simulink library "sim_model_lib"  (R2016b)
settings: Solver=ode45  StartTime=0.0  StopTime=10.0  RelTol=1e-3  EnableMultiTasking=on
libraries: env_environment_model_lib x1, mlp_mid_level_processor_lib x1, veh_vehicle_model_lib x1
settings Model: Creator=jfusco1  LastModifiedBy=jfusco1
settings DataIOCC: LimitDataPoints=on  SaveFormat=Array
settings OptimizationCC: LifeSpan=inf
settings DebuggingCC: SolverPrmCheckMsg=warning  AllowSymbolicDim=off  SFUnexpectedBacktrackingDiag=warning  SFNoUnconditionalDefaultTransitionDiag=warning  SFExecutionAtInitializationDiag=none
settings HardwareCC: ProdBitPerPointer=32  ProdBitPerSizeT=32  ProdBitPerPtrDiffT=32  ProdLargestAtomicFloat=None  ProdIntDivRoundTo=Undefined  ProdEndianess=Unspecified  ProdWordSize=32  ProdHWDeviceType=32-bit Generic
settings ModelReferenceCC: PropagateSignalLabelsOutOfModel=off
settings GRTTargetCC: TargetLangStandard=C89/C90 (ANSI)  GeneratePreprocessorConditionals=Disable all
settings ConfigComp: CovMetricSettings=dw  CovHtmlReporting=on  CovSaveCumulativeToWorkspaceVar=on  CovSaveSingleToWorkspaceVar=on  CovExternalEMLEnable=off  CovSFcnEnable=off

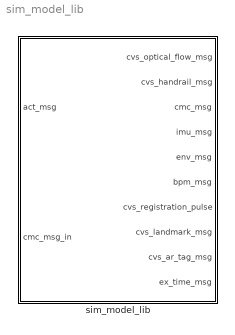
== system sim_model_lib ==
  sim_model_lib : Subsystem

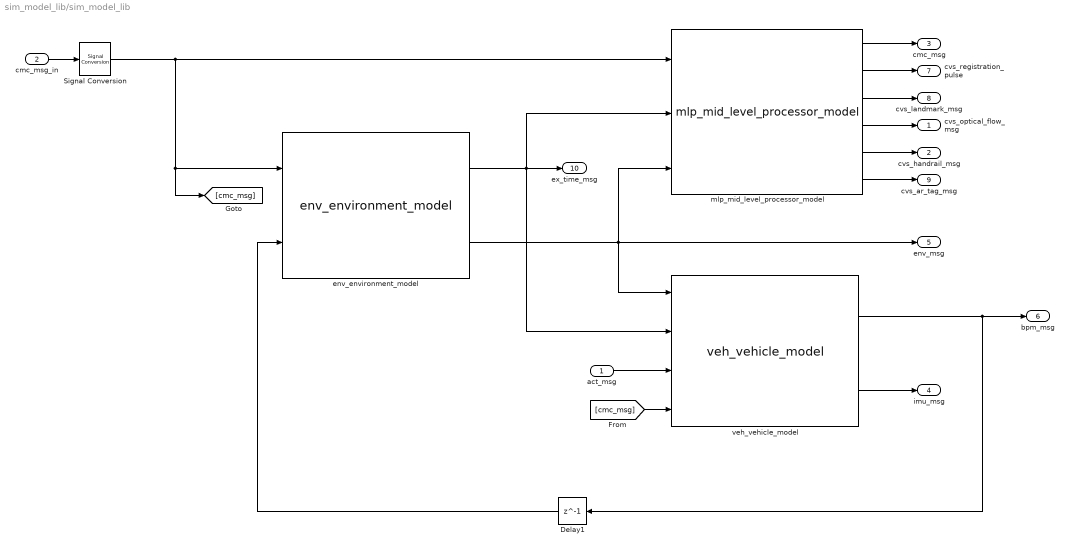
== system sim_model_lib/sim_model_lib ==
  act_msg : Inport  OutDataTypeStr=Bus: act_msg
  cmc_msg_in : Inport  Port=2  OutDataTypeStr=Bus: cmc_msg
  Delay1 : Delay  DelayLength=1
  Signal Conversion : SignalConversion  OverrideOpt=on
  env_environment_model : env_environment_model_lib/env_environment_model  VariantControl=(default)
  mlp_mid_level_processor_model : mlp_mid_level_processor_lib/mlp_mid_level_processor_model
  veh_vehicle_model : veh_vehicle_model_lib/veh_vehicle_model
  cvs_optical_flow_msg : Outport  OutDataTypeStr=Bus: cvs_optical_flow_msg
  cvs_handrail_msg : Outport  Port=2
  cmc_msg : Outport  Port=3  OutDataTypeStr=Bus: cmc_msg
  imu_msg : Outport  Port=4  OutDataTypeStr=Bus: imu_msg
  env_msg : Outport  Port=5  OutDataTypeStr=Bus: env_msg
  bpm_msg : Outport  Port=6
  cvs_registration_pulse : Outport  Port=7  OutDataTypeStr=Bus: cvs_registration_pulse
  cvs_landmark_msg : Outport  Port=8  OutDataTypeStr=Bus: cvs_landmark_msg
  cvs_ar_tag_msg : Outport  Port=9
  ex_time_msg : Outport  Port=10  OutDataTypeStr=Bus: ex_time_msg
  wires:
  mlp_mid_level_processor_model/5 -> cvs_handrail_msg/1
  Delay1/1 -> env_environment_model/2
  act_msg/1 -> veh_vehicle_model/3
  veh_vehicle_model/1 -> Delay1/1, bpm_msg/1
  mlp_mid_level_processor_model/2 -> cvs_registration_pulse/1
  mlp_mid_level_processor_model/3 -> cvs_landmark_msg/1
  env_environment_model/1 -> mlp_mid_level_processor_model/2, ex_time_msg/1, veh_vehicle_model/2
  mlp_mid_level_processor_model/1 -> cmc_msg/1
  mlp_mid_level_processor_model/4 -> cvs_optical_flow_msg/1
  veh_vehicle_model/2 -> imu_msg/1
  env_environment_model/2 -> mlp_mid_level_processor_model/3, env_msg/1, veh_vehicle_model/1
  mlp_mid_level_processor_model/6 -> cvs_ar_tag_msg/1
  Signal Conversion/1 -> mlp_mid_level_processor_model/1, [cmc_msg], env_environment_model/1
  [cmc_msg] -> veh_vehicle_model/4
  cmc_msg_in/1 -> Signal Conversion/1
